simulink model "Copy_of_Robot_PD_Trajectory_Control_"  (R2020b)
settings: Solver=VariableStepAuto  StartTime=0.0  StopTime=6  RelTol=1e-3  EnableMultiTasking=on
model workspace: external: MATLAB File D:\Google Drive\Duongw_Folder\Thesis Master\_Model\Delta_Model_ADEPT\SIMCAPE_MULTI_BODY\ADEPT_DELTA_3AXES1\Assem1_ADEPT_HORNET_DataFile.m (data not in the file)
values from neighbouring files (symbols this model uses):
  G = -5    [Assem1_ADEPT_HORNET_DataFile.m]    (also in data_specMotor.m)
  Kb = 0.4    [Assem1_ADEPT_HORNET_DataFile.m]    (also in data_specMotor.m)
  Km = 0.7    [Assem1_ADEPT_HORNET_DataFile.m]    (also in data_specMotor.m)
  La = 0.0062000000000000006    (= 0.0062)    [Assem1_ADEPT_HORNET_DataFile.m]    (also in data_specMotor.m)
  m = zeros(1,3)    [forward.m]    (also in solequa.m = zeros(3,1))
  Ra = 1.8    [Assem1_ADEPT_HORNET_DataFile.m]    (also in data_specMotor.m)
  smiData = struct    [Assem1_ADEPT_HORNET_DataFile.m]
undefined symbols (not defined in the file or in its folder): X, Y, Z
libraries: sm_lib x106, nesl_utility x7, pid_lib x3
(part 1 of 4)
settings Model: Creator=ThanhUTC  LastModifiedBy=ShiningDanyang
settings SolverCC: ZeroCrossAlgorithm=Adaptive
settings DataIOCC: SaveFormat=Array  ReturnWorkspaceOutputs=off
settings OptimizationCC: LifeSpan=inf
settings DebuggingCC: MaxConsecutiveZCsMsg=none  SFUnexpectedBacktrackingDiag=warning  SFNoUnconditionalDefaultTransitionDiag=warning  SFExecutionAtInitializationDiag=none  ArithmeticOperatorsInVariantConditions=warning
settings SFSimCC: SimUseLocalCustomCode=off  CustomCodeUndefinedFunction=UseInterfaceOnly
settings RTWCC: RTWUseLocalCustomCode=off
settings CodeAppCC: StateflowObjectComments=on
settings GRTTargetCC: TargetLangStandard=C89/C90 (ANSI)
settings ConfigComp: CovMetricSettings=dw  CovSaveCumulativeToWorkspaceVar=on  CovSaveSingleToWorkspaceVar=on  CovExternalEMLEnable=off
settings SimscapeCC: SimscapeNormalizeSystem=off
settings ExplorerConfigSet: InternalSimMechanicsExplorerSettings="<ExplorerConfiguration><canonicalview>aerospace</canonicalview><AnimationSetting><BasePlaybackSpeed>1.0</BasePlaybackSpeed><PlaybackSpeedFactor>1.0</PlaybackSpeedFactor></AnimationSetting><TilePanel><TileInfo><Tiles Columns=\"1\" Count=\"1\" Rows=\"1\"><Column Left=\"2\" Weight=\"1\"/><Column Left=\"948\"/><Row Top=\"2\" Weight=\"1\"/><Row Top=\"599\"/><Tile Height=\"1\" Width=\"1\" X=\"0\" Y=\"0\"/></Tiles></TileInfo><SceneInfo><SceneViewer><BGColor><R>0.60000002384185791</R><G>0.60000002384185791</G><B>0.60000002384185791</B></BGColor><Camera><DoPerspective>off</DoPerspective><Position><X>-0.12822466747721339</X><Y>1.2164090922931379</Y><Z>0.31439967074957181</Z></Position><Center><X>-0.12822466747721339</X><Y>0.15579592814266618</Y><Z>0.31439967074957181</Z></Center><Up><X>0</X><Y>0</Y><Z>-1</Z></Up><ViewLimDist>1</ViewLimDist><YLim>0.98441340628462559</YLim><XLim>1.5686995947086637</XLim></Camera></SceneViewer></SceneInfo></TilePanel><MechEditorPanel><Cameras/><GfxPanelCameraMap/></MechEditorPanel></ExplorerConfiguration>"

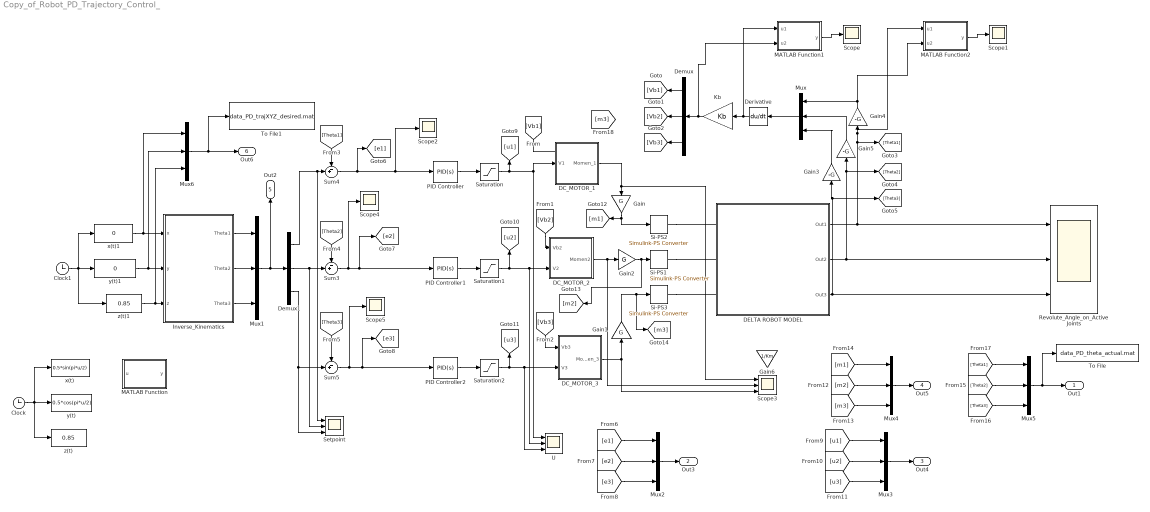
== system Copy_of_Robot_PD_Trajectory_Control_ ==
  Clock : Clock
  Clock1 : Clock
  DC_MOTOR_1 : Subsystem
  DC_MOTOR_2 : Subsystem
  DC_MOTOR_3 : Subsystem
  DELTA ROBOT MODEL : Subsystem
  Demux : Demux  Outputs=3
  Demux1 : Demux  Outputs=3
  Derivative : Derivative
  Gain : Gain  Gain=G
  Gain1 : Gain  Gain=G
  Gain2 : Gain  Gain=G
  Gain3 : Gain  Gain=-G
  Gain4 : Gain  Gain=-G
  Gain5 : Gain  Gain=-G
  Gain6 : Gain  Gain=1/Km
  Inverse_Kinematics : Subsystem
  Kb : Gain  Gain=Kb
  MATLAB Function : MATLAB Function  TreatAsAtomicUnit=on
  MATLAB Function1 : MATLAB Function  TreatAsAtomicUnit=on
  MATLAB Function2 : MATLAB Function  TreatAsAtomicUnit=on
  Mux{,1..6} (7 alike) : Mux  Inputs=3
  PID Controller : pid_lib/PID Controller  Controller=PID  Form=Parallel  TimeDomain=Continuous-time  UseExternalTs=off  SampleTime=-1  IntegratorMethod=Forward Euler  FilterMethod=Forward Euler  ControllerParametersSource=internal  P=300  I=15  D=0  UseFilter=on  N=100  TunerSelectOption=Transfer Function Based (PID Tuner App)  InitialConditionSource=internal  InitialConditionForIntegrator=0  InitialConditionForFilter=0  DifferentiatorICPrevScaledInput=0  ExternalReset=none  TrackingMode=off  Kt=1  LimitOutput=off  SatLimitsSource=internal  UpperSaturationLimit=inf  LowerSaturationLimit=-inf  LinearizeAsGain=on  AntiWindupMode=none  Kb=1  POutMin=[]  POutMax=[]  IOutMin=[]  IOutMax=[]  DOutMin=[]  DOutMax=[]  NOutMin=[]  NOutMax=[]  SumOutMin=[]  SumOutMax=[]  SaturationOutMin=[]  SaturationOutMax=[]  PParamMin=[]  PParamMax=[]  IParamMin=[]  IParamMax=[]  DParamMin=[]  DParamMax=[]  NParamMin=[]  NParamMax=[]  KbParamMin=[]  KbParamMax=[]  KtParamMin=[]  KtParamMax=[]  KbOutMin=[]  KbOutMax=[]  KtOutMin=[]  KtOutMax=[]  IntegratorOutMin=[]  IntegratorOutMax=[]  FilterOutMin=[]  FilterOutMax=[]  SumI1OutMin=[]  SumI1OutMax=[]  SumI2OutMin=[]  SumI2OutMax=[]  SumI3OutMin=[]  SumI3OutMax=[]  SumI4OutMin=[]  SumI4OutMax=[]  SumDOutMin=[]  SumDOutMax=[]  DifferentiatorOutMin=[]  DifferentiatorOutMax=[]  FilterDiffOutCoefMin=[]  FilterDiffOutCoefMax=[]  ReciprocalOutMin=[]  ReciprocalOutMax=[]  SumDenOutMin=[]  SumDenOutMax=[]  SumNumOutMin=[]  SumNumOutMax=[]  DivideOutMin=[]  DivideOutMax=[]  UdiffTsProdOutMin=[]  UdiffTsProdOutMax=[]  NTsProdOutMin=[]  NTsProdOutMax=[]  UintegralTsProdOutMin=[]  UintegralTsProdOutMax=[]  UngainTsProdOutMin=[]  UngainTsProdOutMax=[]  IntegratorContinuousStateAttributes=''  IntegratorStateMustResolveToSignalObject=off  IntegratorRTWStateStorageClass=Auto  FilterContinuousStateAttributes=''  FilterStateMustResolveToSignalObject=off  FilterRTWStateStorageClass=Auto  ParallelPVariant=InternalParameters  IdealPVariant=Disabled  IVariant=InternalParameters  DVariant=InternalParameters  IntegratorVariant=Continuous  SatVariant=Disabled  AWVariant=Passthrough  PCopyVariant=Disabled  TRVariant=Disabled  FdbkBlocksVariant=Forward  IdealPFdbkVariant=Disabled  SatFdbkVariant=Disabled  DerivativeFilterVariant=ContFilter  NVariant=InternalParameters  NCopyVariant=Disabled  FilterICVariant=InternalICsFilter  IntegratorICVariant=InternalICs  ExternalResetVariant=Disabled  TRSumVariant=Passthrough  SumFdbkVariant=Disabled  SumVariant=Sum_PID  TsampFilterVariant=InternalTs  TsampNgainVariant=Passthrough  TsampIntegralVariant=Passthrough  ExternalSaturationOutDataTypeStr=Inherit: Same as second input
  PID Controller1 : pid_lib/PID Controller  Controller=PID  Form=Parallel  TimeDomain=Continuous-time  UseExternalTs=off  SampleTime=-1  IntegratorMethod=Forward Euler  FilterMethod=Forward Euler  ControllerParametersSource=internal  P=300  I=15  D=0  UseFilter=on  N=100  TunerSelectOption=Transfer Function Based (PID Tuner App)  InitialConditionSource=internal  InitialConditionForIntegrator=0  InitialConditionForFilter=0  DifferentiatorICPrevScaledInput=0  ExternalReset=none  TrackingMode=off  Kt=1  LimitOutput=off  SatLimitsSource=internal  UpperSaturationLimit=inf  LowerSaturationLimit=-inf  LinearizeAsGain=on  AntiWindupMode=none  Kb=1  POutMin=[]  POutMax=[]  IOutMin=[]  IOutMax=[]  DOutMin=[]  DOutMax=[]  NOutMin=[]  NOutMax=[]  SumOutMin=[]  SumOutMax=[]  SaturationOutMin=[]  SaturationOutMax=[]  PParamMin=[]  PParamMax=[]  IParamMin=[]  IParamMax=[]  DParamMin=[]  DParamMax=[]  NParamMin=[]  NParamMax=[]  KbParamMin=[]  KbParamMax=[]  KtParamMin=[]  KtParamMax=[]  KbOutMin=[]  KbOutMax=[]  KtOutMin=[]  KtOutMax=[]  IntegratorOutMin=[]  IntegratorOutMax=[]  FilterOutMin=[]  FilterOutMax=[]  SumI1OutMin=[]  SumI1OutMax=[]  SumI2OutMin=[]  SumI2OutMax=[]  SumI3OutMin=[]  SumI3OutMax=[]  SumI4OutMin=[]  SumI4OutMax=[]  SumDOutMin=[]  SumDOutMax=[]  DifferentiatorOutMin=[]  DifferentiatorOutMax=[]  FilterDiffOutCoefMin=[]  FilterDiffOutCoefMax=[]  ReciprocalOutMin=[]  ReciprocalOutMax=[]  SumDenOutMin=[]  SumDenOutMax=[]  SumNumOutMin=[]  SumNumOutMax=[]  DivideOutMin=[]  DivideOutMax=[]  UdiffTsProdOutMin=[]  UdiffTsProdOutMax=[]  NTsProdOutMin=[]  NTsProdOutMax=[]  UintegralTsProdOutMin=[]  UintegralTsProdOutMax=[]  UngainTsProdOutMin=[]  UngainTsProdOutMax=[]  IntegratorContinuousStateAttributes=''  IntegratorStateMustResolveToSignalObject=off  IntegratorRTWStateStorageClass=Auto  FilterContinuousStateAttributes=''  FilterStateMustResolveToSignalObject=off  FilterRTWStateStorageClass=Auto  ParallelPVariant=InternalParameters  IdealPVariant=Disabled  IVariant=InternalParameters  DVariant=InternalParameters  IntegratorVariant=Continuous  SatVariant=Disabled  AWVariant=Passthrough  PCopyVariant=Disabled  TRVariant=Disabled  FdbkBlocksVariant=Forward  IdealPFdbkVariant=Disabled  SatFdbkVariant=Disabled  DerivativeFilterVariant=ContFilter  NVariant=InternalParameters  NCopyVariant=Disabled  FilterICVariant=InternalICsFilter  IntegratorICVariant=InternalICs  ExternalResetVariant=Disabled  TRSumVariant=Passthrough  SumFdbkVariant=Disabled  SumVariant=Sum_PID  TsampFilterVariant=InternalTs  TsampNgainVariant=Passthrough  TsampIntegralVariant=Passthrough  ExternalSaturationOutDataTypeStr=Inherit: Same as second input
  PID Controller2 : pid_lib/PID Controller  Controller=PID  Form=Parallel  TimeDomain=Continuous-time  UseExternalTs=off  SampleTime=-1  IntegratorMethod=Forward Euler  FilterMethod=Forward Euler  ControllerParametersSource=internal  P=300  I=15  D=0  UseFilter=on  N=100  TunerSelectOption=Transfer Function Based (PID Tuner App)  InitialConditionSource=internal  InitialConditionForIntegrator=0  InitialConditionForFilter=0  DifferentiatorICPrevScaledInput=0  ExternalReset=none  TrackingMode=off  Kt=1  LimitOutput=off  SatLimitsSource=internal  UpperSaturationLimit=inf  LowerSaturationLimit=-inf  LinearizeAsGain=on  AntiWindupMode=none  Kb=1  POutMin=[]  POutMax=[]  IOutMin=[]  IOutMax=[]  DOutMin=[]  DOutMax=[]  NOutMin=[]  NOutMax=[]  SumOutMin=[]  SumOutMax=[]  SaturationOutMin=[]  SaturationOutMax=[]  PParamMin=[]  PParamMax=[]  IParamMin=[]  IParamMax=[]  DParamMin=[]  DParamMax=[]  NParamMin=[]  NParamMax=[]  KbParamMin=[]  KbParamMax=[]  KtParamMin=[]  KtParamMax=[]  KbOutMin=[]  KbOutMax=[]  KtOutMin=[]  KtOutMax=[]  IntegratorOutMin=[]  IntegratorOutMax=[]  FilterOutMin=[]  FilterOutMax=[]  SumI1OutMin=[]  SumI1OutMax=[]  SumI2OutMin=[]  SumI2OutMax=[]  SumI3OutMin=[]  SumI3OutMax=[]  SumI4OutMin=[]  SumI4OutMax=[]  SumDOutMin=[]  SumDOutMax=[]  DifferentiatorOutMin=[]  DifferentiatorOutMax=[]  FilterDiffOutCoefMin=[]  FilterDiffOutCoefMax=[]  ReciprocalOutMin=[]  ReciprocalOutMax=[]  SumDenOutMin=[]  SumDenOutMax=[]  SumNumOutMin=[]  SumNumOutMax=[]  DivideOutMin=[]  DivideOutMax=[]  UdiffTsProdOutMin=[]  UdiffTsProdOutMax=[]  NTsProdOutMin=[]  NTsProdOutMax=[]  UintegralTsProdOutMin=[]  UintegralTsProdOutMax=[]  UngainTsProdOutMin=[]  UngainTsProdOutMax=[]  IntegratorContinuousStateAttributes=''  IntegratorStateMustResolveToSignalObject=off  IntegratorRTWStateStorageClass=Auto  FilterContinuousStateAttributes=''  FilterStateMustResolveToSignalObject=off  FilterRTWStateStorageClass=Auto  ParallelPVariant=InternalParameters  IdealPVariant=Disabled  IVariant=InternalParameters  DVariant=InternalParameters  IntegratorVariant=Continuous  SatVariant=Disabled  AWVariant=Passthrough  PCopyVariant=Disabled  TRVariant=Disabled  FdbkBlocksVariant=Forward  IdealPFdbkVariant=Disabled  SatFdbkVariant=Disabled  DerivativeFilterVariant=ContFilter  NVariant=InternalParameters  NCopyVariant=Disabled  FilterICVariant=InternalICsFilter  IntegratorICVariant=InternalICs  ExternalResetVariant=Disabled  TRSumVariant=Passthrough  SumFdbkVariant=Disabled  SumVariant=Sum_PID  TsampFilterVariant=InternalTs  TsampNgainVariant=Passthrough  TsampIntegralVariant=Passthrough  ExternalSaturationOutDataTypeStr=Inherit: Same as second input
  Revolute_Angle_on_Active Joints : Scope  NumInputPorts=3
  Saturation : Saturate  UpperLimit=24  LowerLimit=-24
  Saturation1 : Saturate  UpperLimit=24  LowerLimit=-24
  Saturation2 : Saturate  UpperLimit=24  LowerLimit=-24
  Scope{,1..2,4..5} (5 alike) : Scope
  Scope3 : Scope  NumInputPorts=3
  Setpoint : Scope  NumInputPorts=3
  Si-PS1 : nesl_utility/Simulink-PS Converter  PhysicalDomain=network_engine_domain  SubClassName=ps_input  LeftPortType=input  RightPortType=output  PseudoPeriodic=off  Frequencies=[]  NoiseDistribution=none  NoiseParameters=[]  Unit=1  AffineConversion=off  FilteringAndDerivatives=filter  SimscapeFilterOrder=2  InputFilterTimeConstant=0.001  UdotUserProvided=1
  Si-PS2 : nesl_utility/Simulink-PS Converter  PhysicalDomain=network_engine_domain  SubClassName=ps_input  LeftPortType=input  RightPortType=output  PseudoPeriodic=off  Frequencies=[]  NoiseDistribution=none  NoiseParameters=[]  Unit=1  AffineConversion=off  FilteringAndDerivatives=filter  SimscapeFilterOrder=2  InputFilterTimeConstant=0.001  UdotUserProvided=1
  Si-PS3 : nesl_utility/Simulink-PS Converter  PhysicalDomain=network_engine_domain  SubClassName=ps_input  LeftPortType=input  RightPortType=output  PseudoPeriodic=off  Frequencies=[]  NoiseDistribution=none  NoiseParameters=[]  Unit=1  AffineConversion=off  FilteringAndDerivatives=filter  SimscapeFilterOrder=2  InputFilterTimeConstant=0.001  UdotUserProvided=1
  Sum3 : Sum  Inputs=-+|
  Sum4 : Sum  Inputs=-+|
  Sum5 : Sum  Inputs=-+|
  To File : ToFile  Filename=data_PD_theta_actual.mat  MatrixName=theta_actual
  To File1 : ToFile  Filename=data_PD_trajXYZ_desired.mat  MatrixName=xyz_d
  "U " : Scope  NumInputPorts=3
  x(t) : Fcn  Expr=0.5*sin(pi*u/2)
  x(t)1 : Fcn  Expr=0
  y(t) : Fcn  Expr=0.5*cos(pi*u/2)
  y(t)1 : Fcn  Expr=0
  z(t) : Fcn  Expr=0.85
  z(t)1 : Fcn  Expr=0.85
  Out1 : Outport  VectorParamsAs1DForOutWhenUnconnected=off
  Out3 : Outport  Port=2  VectorParamsAs1DForOutWhenUnconnected=off
  Out4 : Outport  Port=3  VectorParamsAs1DForOutWhenUnconnected=off
  Out5 : Outport  Port=4  VectorParamsAs1DForOutWhenUnconnected=off
  Out2 : Outport  Port=5  VectorParamsAs1DForOutWhenUnconnected=off
  Out6 : Outport  Port=6  VectorParamsAs1DForOutWhenUnconnected=off
  wires:
  DELTA ROBOT MODEL/2(Out2) -> Gain5/1, [Theta2], Revolute_Angle_on_Active Joints/2
  DELTA ROBOT MODEL/3(Out3) -> Gain3/1, [Theta3], Revolute_Angle_on_Active Joints/3
  Demux/1 -> [Vb1]
  Demux/2 -> [Vb2]
  Demux/3 -> [Vb3]
  [Theta1] -> Sum4/1
  Sum4/1 -> [e1], PID Controller/1, Scope2/1
  [Vb1] -> ?
  PID Controller/1 -> Saturation/1
  [Theta2] -> Sum3/1
  Sum3/1 -> Scope4/1, PID Controller1/1, [e2]
  PID Controller1/1 -> Saturation1/1
  [Theta3] -> Sum5/1
  Sum5/1 -> Scope5/1, PID Controller2/1, [e3]
  PID Controller2/1 -> Saturation2/1
  [Vb2] -> DC_MOTOR_2/1(Vb2)
  [Vb3] -> DC_MOTOR_3/1(Vb3)
  Gain/1 -> [m1], Si-PS2/1
  Gain1/1 -> [m3], Si-PS3/1
  Gain2/1 -> [m2], Si-PS1/1
  Saturation/1 -> [u1], DC_MOTOR_1/1(V1), "U "/1
  Saturation1/1 -> [u2], "U "/2, DC_MOTOR_2/2(V2)
  Saturation2/1 -> [u3], "U "/3, DC_MOTOR_3/2(V3)
  Gain3/1 -> Mux/3
  Gain5/1 -> Mux/2
  Mux/1 -> Derivative/1
  Demux1/1 -> Setpoint/1, Sum4/2
  Demux1/2 -> Setpoint/2, Sum3/2
  Demux1/3 -> Setpoint/3, Sum5/2
  [e1] -> Mux2/1
  [e2] -> Mux2/2
  [e3] -> Mux2/3
  [u1] -> Mux3/1
  [u2] -> Mux3/2
  [u3] -> Mux3/3
  Mux2/1 -> Out3/1
  Mux3/1 -> Out4/1
  [m1] -> Mux4/1
  [m2] -> Mux4/2
  [m3] -> Mux4/3
  Mux4/1 -> Out5/1
  [Theta1] -> Mux5/1
  [Theta2] -> Mux5/2
  [Theta3] -> Mux5/3
  x(t)1/1 -> Mux6/1, Inverse_Kinematics/1(x)
  y(t)1/1 -> Mux6/2, Inverse_Kinematics/2(y)
  Inverse_Kinematics/1(Theta1) -> Mux1/1
  Inverse_Kinematics/2(Theta2) -> Mux1/2
  Inverse_Kinematics/3(Theta3) -> Mux1/3
  Mux1/1 -> Demux1/1, Out2/1
  Mux5/1 -> To File/1, Out1/1
  Mux6/1 -> To File1/1, Out6/1
  z(t)1/1 -> Mux6/3, Inverse_Kinematics/3(z)
  Clock/1 -> z(t)/1, x(t)/1, y(t)/1
  Clock1/1 -> z(t)1/1, x(t)1/1, y(t)1/1
  DC_MOTOR_1/1(Momen_1) -> Scope3/1, Gain/1
  DC_MOTOR_2/1(Momen2) -> Scope3/2, Gain2/1
  DC_MOTOR_3/1(Momen_3) -> Scope3/3, Gain1/1
  Derivative/1 -> MATLAB Function1/1(u1), Kb/1
  MATLAB Function1/1(y) -> Scope/1
  Kb/1 -> MATLAB Function1/2(u2), Demux/1
  DELTA ROBOT MODEL/1(Out1) -> MATLAB Function2/1(u1), Gain4/1, [Theta1], Revolute_Angle_on_Active Joints/1
  Gain4/1 -> MATLAB Function2/2(u2), Mux/1
  MATLAB Function2/1(y) -> Scope1/1
  connections:
  Si-PS2/RConn1 -- DELTA ROBOT MODEL/LConn1
  Si-PS1/RConn1 -- DELTA ROBOT MODEL/LConn2
  Si-PS3/RConn1 -- DELTA ROBOT MODEL/LConn3

== system Copy_of_Robot_PD_Trajectory_Control_/DC_MOTOR_1 ==
  V1 : Inport
  Gain1 : Gain  Gain=Km
  Transfer Fcn : TransferFcn  Denominator=[La Ra]
  Momen_1 : Outport  VectorParamsAs1DForOutWhenUnconnected=off
  wires:
  V1/1 -> Transfer Fcn/1
  Transfer Fcn/1 -> Gain1/1
  Gain1/1 -> Momen_1/1

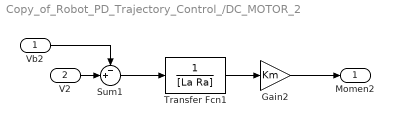
== system Copy_of_Robot_PD_Trajectory_Control_/DC_MOTOR_2 ==
  Vb2 : Inport
  V2 : Inport  Port=2
  Gain2 : Gain  Gain=Km
  Sum1 : Sum  Inputs=-+|
  Transfer Fcn1 : TransferFcn  Denominator=[La Ra]
  Momen2 : Outport  VectorParamsAs1DForOutWhenUnconnected=off
  wires:
  Vb2/1 -> Sum1/1
  Transfer Fcn1/1 -> Gain2/1
  Sum1/1 -> Transfer Fcn1/1
  Gain2/1 -> Momen2/1
  V2/1 -> Sum1/2

== system Copy_of_Robot_PD_Trajectory_Control_/DC_MOTOR_3 ==
  Vb3 : Inport
  V3 : Inport  Port=2
  Gain3 : Gain  Gain=Km
  Sum2 : Sum  Inputs=-+|
  Transfer Fcn2 : TransferFcn  Denominator=[La Ra]
  Momen_3 : Outport  VectorParamsAs1DForOutWhenUnconnected=off
  wires:
  Vb3/1 -> Sum2/1
  Transfer Fcn2/1 -> Gain3/1
  Sum2/1 -> Transfer Fcn2/1
  Gain3/1 -> Momen_3/1
  V3/1 -> Sum2/2
